simulink model "pendrag"  (Simulink 4.00)
settings: Solver=ode45  StartTime=0.0  StopTime=10  RelTol=1e-3
values from neighbouring files (symbols this model uses):
  g = 9.81    [cannonballpar.m]    (also in pendcartpar.m = 1; pendragpar.m)
  kappa = rho*S*Cd/2    (= 0.007618)    [cannonballpar.m]    (also in pendragpar.m = 0.0003809)
  l = 1    [pend4par.m]    (also in pendcartpar.m; pendragpar.m = 0.1)
  m = 1    [cannonballpar.m]    (also in pendcartpar.m; pendragpar.m = 0.01)
  w = 1    [pendragpar.m]

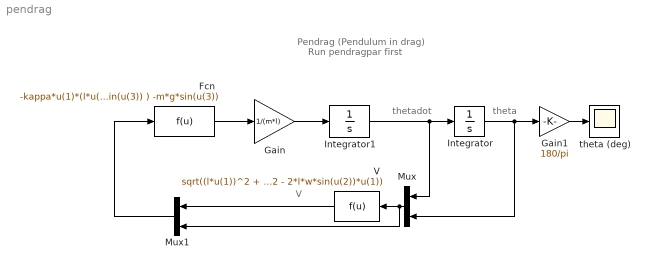
== system pendrag ==
  note: thetadot
  note: theta
  note: Pendrag (Pendulum in drag)
  note: Run pendragpar first
  note: V
  Fcn : Fcn  Expr=-kappa*u(1)*(l*u(2)-w*sin(u(3)) ) -m*g*sin(u(3))
  Gain : Gain  Gain=1/(m*l)  Multiplication=Element-wise(K.*u)  SaturateOnIntegerOverflow=on
  Gain1 : Gain  Gain=180/pi  Multiplication=Element-wise(K.*u)  SaturateOnIntegerOverflow=on
  Integrator : Integrator  ExternalReset=none  InitialConditionSource=internal  InitialCondition=45*pi/180  LimitOutput=off  UpperSaturationLimit=inf  LowerSaturationLimit=-inf  ShowSaturationPort=off  ShowStatePort=off  AbsoluteTolerance=auto
  Integrator1 : Integrator  ExternalReset=none  InitialConditionSource=internal  InitialCondition=0  LimitOutput=off  UpperSaturationLimit=inf  LowerSaturationLimit=-inf  ShowSaturationPort=off  ShowStatePort=off  AbsoluteTolerance=auto
  Mux : Mux  Orientation=left  Inputs=2
  Mux1 : Mux  Orientation=left  Inputs=2
  V : Fcn  Orientation=left  Expr=sqrt((l*u(1))^2 + w^2 - 2*l*w*sin(u(2))*u(1))
  theta (deg) : Scope
      settings: TimeRange=auto  YMin=-5  YMax=5  SaveToWorkspace=off  SaveName=ScopeData  LimitDataPoints=on  MaxDataPoints=5000
  wires:
  Integrator1/1 -> Integrator/1, Mux/1
  Integrator/1 -> Mux/2, Gain1/1
  Mux/1 -> V/1, Mux1/2
  V/1 -> Mux1/1
  Gain/1 -> Integrator1/1
  Mux1/1 -> Fcn/1
  Fcn/1 -> Gain/1
  Gain1/1 -> theta (deg)/1
